simulink model "match_141121"  (R2018b)
settings: Solver=FixedStepDiscrete  StartTime=0.0  StopTime=1  RelTol=1e-3
undefined symbols (not defined in the file or in its folder): gray
libraries: hdlsllib x6, visionsources x1, dspmtrx3 x1
settings Model: Creator=Administrator  LastModifiedBy=Administrator
settings OptimizationCC: BlockReduction=off  ConditionallyExecuteInputs=off  DefaultParameterBehavior=Inlined
settings DebuggingCC: AlgebraicLoopMsg=error  SingleTaskRateTransMsg=error
settings HardwareCC: ProdBitPerPointer=32  ProdBitPerSizeT=32  ProdBitPerPtrDiffT=32  ProdLargestAtomicFloat=None  ProdIntDivRoundTo=Undefined  ProdEndianess=Unspecified  ProdWordSize=32  ProdHWDeviceType=ASIC/FPGA->ASIC/FPGA  TargetBitPerPointer=64  TargetBitPerSizeT=64  TargetBitPerPtrDiffT=64  TargetLongLongMode=on  TargetIntDivRoundTo=Zero  TargetEndianess=LittleEndian  TargetWordSize=64  TargetHWDeviceType=Custom Processor->MATLAB Host Computer  ProdEqTarget=off

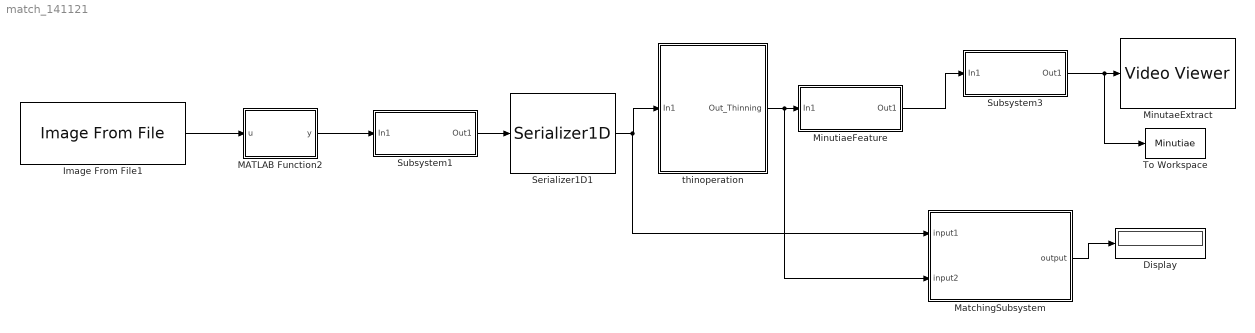
== system match_141121 ==
  Display : Display
  Image From File1 : visionsources/Image From File  Tag=vipblks_nd  FileName=C:\Users\Administrator\Desktop\chapter\101_4.tif  imagePorts=One multidimensional signal  Ts=0.1  ImageDataType=uint8  Signed=on  WordLength=16  sdImageDataType=uint(8)  FractionLengthMode=User-defined  FractionLength=15  OutPortLabels=R|G|B
      settings: SourceProductName=Computer Vision System Toolbox
  MATLAB Function2 : MATLAB Function  TreatAsAtomicUnit=on
  MatchingSubsystem : Subsystem
  MinutaeExtract : VideoViewer  colormapValue=gray(256)  FigPos=[1 1158 1920 1059]
  MinutiaeFeature : Subsystem  TreatAsAtomicUnit=on
  Serializer1D1 : hdlsllib/HDL Operations/Serializer1D  Ratio=1  IdleCycles=0  validIn=off  startOut=off  validOut=off  inputDataDimensions=8192  inputSampleTime=-1  inputSignalType=auto
      settings: SourceProductName=HDL Coder  SourceProductBaseCode=HD
  Subsystem1 : Subsystem
  Subsystem3 : Subsystem
  To Workspace : ToWorkspace  VariableName=Minutiae  SampleTime=-1
      settings: Save2DSignal=2-D array (concatenate along first dimension)
  thinoperation : Subsystem  TreatAsAtomicUnit=on
  wires:
  MATLAB Function2/1(y) -> Subsystem1/1(In1)
  Image From File1/1 -> MATLAB Function2/1(u)
  Subsystem1/1(Out1) -> Serializer1D1/1
  MinutiaeFeature/1(Out1) -> Subsystem3/1(In1)
  Subsystem3/1(Out1) -> To Workspace/1, MinutaeExtract/1
  Serializer1D1/1 -> MatchingSubsystem/1(input1), thinoperation/1(In1)
  thinoperation/1(Out_Thinning) -> MatchingSubsystem/2(input2), MinutiaeFeature/1(In1)
  MatchingSubsystem/1(output) -> Display/1

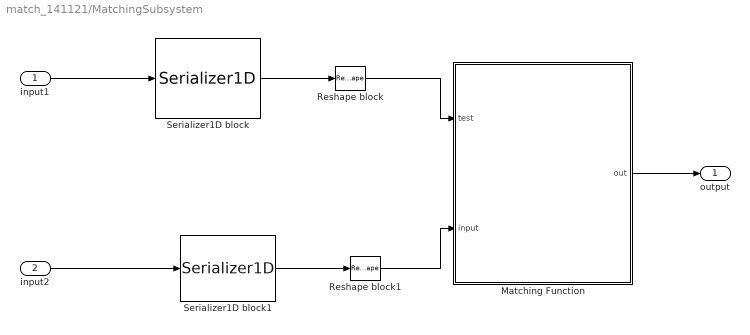
== system match_141121/MatchingSubsystem ==
  input1 : Inport
  input2 : Inport  Port=2
  Matching Function : MATLAB Function  TreatAsAtomicUnit=on
  Reshape block : Reshape  OutputDimensionality=Customize  OutputDimensions=[128,64]
  Reshape block1 : Reshape  OutputDimensionality=Customize  OutputDimensions=[128,64]
  Serializer1D block : hdlsllib/HDL Operations/Serializer1D  Ratio=1  IdleCycles=0  validIn=off  startOut=off  validOut=off  inputDataDimensions=8192  inputSampleTime=-1  inputSignalType=auto
      settings: SourceProductName=HDL Coder  SourceProductBaseCode=HD
  Serializer1D block1 : hdlsllib/HDL Operations/Serializer1D  Ratio=1  IdleCycles=0  validIn=off  startOut=off  validOut=off  inputDataDimensions=8192  inputSampleTime=-1  inputSignalType=auto
      settings: SourceProductName=HDL Coder  SourceProductBaseCode=HD
  output : Outport
  wires:
  Matching Function/1(out) -> output/1
  Serializer1D block/1 -> Reshape block/1
  Reshape block/1 -> Matching Function/1(test)
  input1/1 -> Serializer1D block/1
  Reshape block1/1 -> Matching Function/2(input)
  Serializer1D block1/1 -> Reshape block1/1
  input2/1 -> Serializer1D block1/1

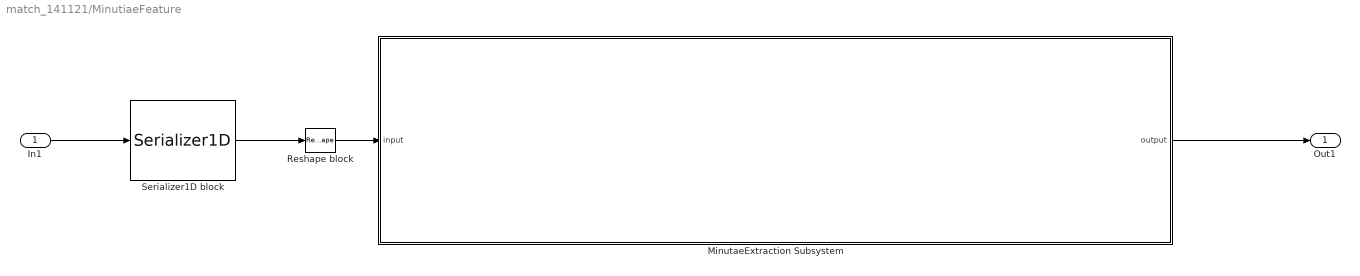
== system match_141121/MinutiaeFeature ==
  In1 : Inport
  MinutaeExtraction Subsystem : Subsystem  TreatAsAtomicUnit=on
  Reshape block : Reshape  OutputDimensionality=Customize  OutputDimensions=[128,64]
  Serializer1D block : hdlsllib/HDL Operations/Serializer1D  Ratio=1  IdleCycles=0  validIn=off  startOut=off  validOut=off  inputDataDimensions=8192  inputSampleTime=-1  inputSignalType=auto
      settings: SourceProductName=HDL Coder  SourceProductBaseCode=HD
  Out1 : Outport
  wires:
  In1/1 -> Serializer1D block/1
  MinutaeExtraction Subsystem/1(output) -> Out1/1
  Reshape block/1 -> MinutaeExtraction Subsystem/1(input)
  Serializer1D block/1 -> Reshape block/1

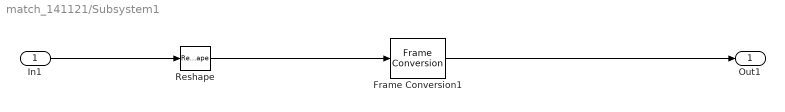
== system match_141121/Subsystem1 ==
  In1 : Inport
  Frame Conversion1 : FrameConversion  OutFrame=Sample-based
  Reshape : Reshape
  Out1 : Outport
  wires:
  Frame Conversion1/1 -> Out1/1
  Reshape/1 -> Frame Conversion1/1
  In1/1 -> Reshape/1

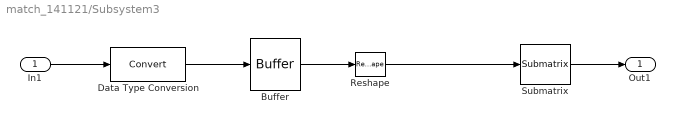
== system match_141121/Subsystem3 ==
  In1 : Inport
  Buffer : Buffer  N=8192  OutputFrames=off
  Data Type Conversion : DataTypeConversion
  Reshape : Reshape  OutputDimensionality=Customize  OutputDimensions=[128,64]
  Submatrix : dspmtrx3/Submatrix  RowSpan=Range of rows  RowStartMode=First  RowStartIndex=1  RowEndMode=Last  RowEndIndex=1  ColSpan=Range of columns  ColStartMode=First  ColStartIndex=1  ColEndMode=Last  ColEndIndex=1
  Out1 : Outport
  wires:
  Data Type Conversion/1 -> Buffer/1
  Buffer/1 -> Reshape/1
  Reshape/1 -> Submatrix/1
  Submatrix/1 -> Out1/1
  In1/1 -> Data Type Conversion/1

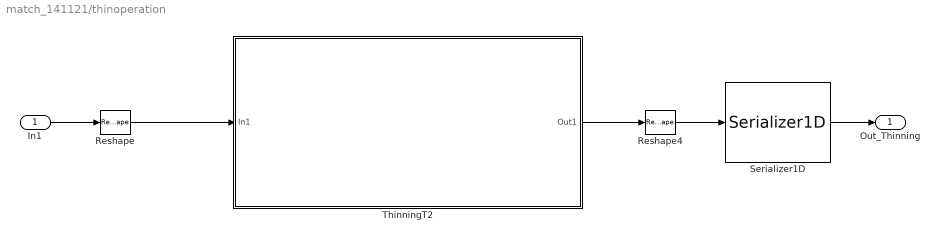
== system match_141121/thinoperation ==
  In1 : Inport
  Reshape : Reshape  OutputDimensionality=Customize  OutputDimensions=[128,64]
  Reshape4 : Reshape  OutputDimensionality=Column vector (2-D)  OutputDimensions=[128,64]
  Serializer1D : hdlsllib/HDL Operations/Serializer1D  Ratio=1  IdleCycles=0  validIn=off  startOut=off  validOut=off  inputDataDimensions=-1  inputSampleTime=-1  inputSignalType=auto
      settings: SourceProductName=HDL Coder  SourceProductBaseCode=HD
  ThinningT2 : Subsystem  TreatAsAtomicUnit=on
  Out_Thinning : Outport
  wires:
  ThinningT2/1(Out1) -> Reshape4/1
  Reshape/1 -> ThinningT2/1(In1)
  Serializer1D/1 -> Out_Thinning/1
  In1/1 -> Reshape/1
  Reshape4/1 -> Serializer1D/1

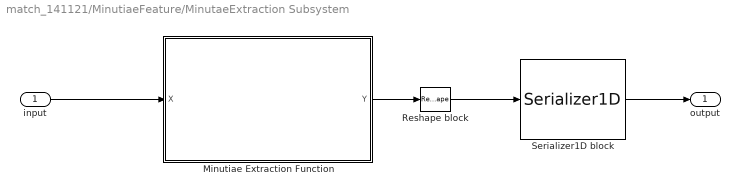
== system match_141121/MinutiaeFeature/MinutaeExtraction Subsystem ==
  input : Inport
  Minutiae Extraction Function : MATLAB Function  TreatAsAtomicUnit=on
  Reshape block : Reshape  OutputDimensionality=Column vector (2-D)  OutputDimensions=[128,64]
  Serializer1D block : hdlsllib/HDL Operations/Serializer1D  Ratio=8192  IdleCycles=0  validIn=off  startOut=off  validOut=off  inputDataDimensions=-1  inputSampleTime=-1  inputSignalType=auto
      settings: SourceProductName=HDL Coder  SourceProductBaseCode=HD
  output : Outport
  wires:
  input/1 -> Minutiae Extraction Function/1(X)
  Serializer1D block/1 -> output/1
  Minutiae Extraction Function/1(Y) -> Reshape block/1
  Reshape block/1 -> Serializer1D block/1

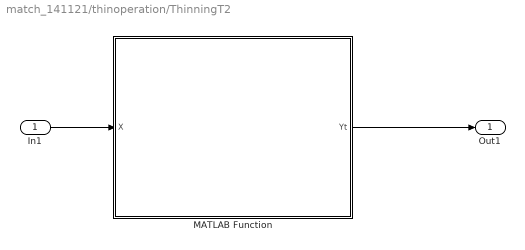
== system match_141121/thinoperation/ThinningT2 ==
  In1 : Inport
  MATLAB Function : MATLAB Function  TreatAsAtomicUnit=on
  Out1 : Outport
  wires:
  In1/1 -> MATLAB Function/1(X)
  MATLAB Function/1(Yt) -> Out1/1

== matlab function match_141121/MATLAB Function2 ==
  data: u input; y output
function y = fcn(u)
%#codegen
%i = rgb2gray(u);
b = u(100:227,150:213);
y = imbinarize(b);
%y = y(100:227,150:213);
%y = imbinarize(r);

== matlab function match_141121/thinoperation/ThinningT2/MATLAB Function ==
  data: X input; Yt output
function Yt=thinningTh(X)
%img = imread ('2_4.jpg'); 
%Xr = rgb2gray(img);
%%%X = imbinarize(Xr);
%X = X(1:128,1:64);
[M,N]=size(X);
Yt = false(M,N);
Y=false(M,N,20);
Z=false(M,N,20);
Y(:,:,1)=X;
Z(:,:,1)=X;
for k=2:20
    Y(:,:,k)=Y(:,:,k-1);
    for i=2:M-1
        for j=2:N-1
            y11=Y(i-1,j-1,k);
            y12=Y(i-1,j,k);
            y13=Y(i-1,j+1,k);
            y21=Y(i,j-1,k);
            y22=Y(i,j,k);
            y23=Y(i,j+1,k);
            y31=Y(i+1,j-1,k);
            y32=Y(i+1,j,k);
            y33=Y(i+1,j+1,k);
            if y22==0
                if y11==1&&y12==1&&y13==1&&y31==0&&y32==0&&y33==0
                    Y(i,j,k)=1;
                elseif y11==1&&y13==0&&y21==1&&y23==0&&y31==1&&y33==0
                    Y(i,j,k)=1;
                elseif y11==0&&y12==0&&y13==0&&y31==1&&y32==1&&y33==1
                    Y(i,j,k)=1;
                elseif y11==0&&y13==1&&y21==0&&y23==1&&y31==0&&y33==1
                    Y(i,j,k)=1;
                elseif y12==1&&y13==1&&y21==0&&y23==1&&y32==0
                    Y(i,j,k)=1;
                elseif y11==1&&y12==1&&y21==1&&y23==0&&y32==0
                    Y(i,j,k)=1;
                elseif y12==0&&y21==1&&y23==0&&y31==1&&y21==1
                    Y(i,j,k)=1;
                elseif y12==0&&y21==0&&y23==1&&y32==1&&y33==1
                    Y(i,j,k)=1;
                    %extra
                elseif y11==0&&y12==0&&y23==1&&y31==1&&y32==1&&y33==1
                    Y(i,j,k)=1;
                end
            else
            end
        end
    end
%    Y(:,:,k)= Y(:,:,k-1);
     if Y(:,:,k)==Y(:,:,k-1)
%         break;
     end
end
Yt=Y(:,:,k);
%figure;
%imshow(Y);

== matlab function match_141121/MatchingSubsystem/Matching Function ==
  data: test input; out output; input input
function out = match(test, input)
%test = zeros(rows,col);
%input = zeros(rows,col);
%[row,col]= size(input);
test = uint8(test);
input = uint8(input);
for i=1:128
    for j=1:64
        %input(i,j);
        if test == input
            out = 1;
        else
            out = 0;
        end
    end
end
end

== matlab function match_141121/MinutiaeFeature/MinutaeExtraction Subsystem/Minutiae Extraction Function ==
  data: X input; Y output
function Y=minuextractT(X)
%img = imread ('101_7.tif'); 
%Xr = rgb2gray(img);
%Xt = imbinarize(img);
%X=~bwmorph(Xt,'thin',Inf);
[M,N]=size(X);
%mi(:,:)=X;
Y=false(M,N);
Y(:,:)=X;
%[M,N]=size(X);
mi=false(M,N);

for i=2:M-1
    for j=2:N-1
        % * * * y11 y12 y13
        % * @ * y21 y22 y23
        % * * * y31 y32 y33
        y11=Y(i-1,j-1);
        y12=Y(i-1,j);
        y13=Y(i-1,j+1);
        y21=Y(i,j-1);
        y22=Y(i,j);
        y23=Y(i,j+1);
        y31=Y(i+1,j-1);
        y32=Y(i+1,j);
        y33=Y(i+1,j+1);
        if y22==0
            if y11+y12+y13+y23+y33+y31+y21+y32==7
                mi(i,j)=1;
            elseif y11==0 && y12==1 && y13==0 && y21==1 && y23==1 && y31==1 && y32==0 && y33==1
                mi(i,j)=2;
            elseif y11==1 && y12==0 && y13==1 && y21==1 && y23==1 && y31==0 && y32==1 && y33==0
                mi(i,j)=2;
            elseif y11==0 && y12==1 && y13==1 && y21==1 && y23==0 && y31==0 && y32==1 && y33==1
                mi(i,j)=2;
            elseif y11==1 && y12==1 && y13==0 && y21==0 && y23==1 && y31==1 && y32==1 && y33==0
                mi(i,j)=2;
            elseif y11==1 && y12==0 && y13==1 && y21==0 && y23==0 && y31==1 && y32==1 && y33==1
                mi(i,j)=2;
            elseif y11==1 && y12==1 && y13==1 && y21==0 && y23==0 && y31==1 && y32==0 && y33==1
                mi(i,j)=2;
            elseif y11==1 && y12==0 && y13==1 && y21==0 && y23==1 && y31==1 && y32==0 && y33==1
                mi(i,j)=2;
            elseif y11==1 && y12==0 && y13==1 && y21==1 && y23==0 && y31==1 && y32==0 && y33==1
                mi(i,j)=2;
            elseif y11==0 && y12==1 && y13==0 && y21==1 && y23==1 && y31==0 && y32==1 && y33==1
                mi(i,j)=2;
            elseif y11==0 && y12==1 && y13==1 && y21==1 && y23==1 && y31==0 && y32==1 && y33==0
                mi(i,j)=2;
            elseif y11==0 && y12==1 && y13==0 && y21==1 && y23==1 && y31==1 && y32==1 && y33==0
                mi(i,j)=2;
            elseif y11==1 && y12==1 && y13==0 && y21==1 && y23==1 && y31==0 && y32==1 && y33==0
                mi(i,j)=2;
            elseif y11==1 && y12==0 && y13==1 && y21==0 && y23==0 && y31==0 && y32==1 && y33==1
                mi(i,j)=2;
            elseif y11==1 && y12==0 && y13==1 && y21==0 && y23==0 && y31==1 && y32==1 && y33==0
                mi(i,j)=2;
            elseif y11==0 && y12==1 && y13==1 && y21==0 && y23==0 && y31==1 && y32==0 && y33==1
                mi(i,j)=2;
            elseif y11==1 && y12==1 && y13==0 && y21==0 && y23==0 && y31==1 && y32==0 && y33==1
                mi(i,j)=2;
            elseif y11==1 && y12==1 && y13==0 && y21==0 && y23==1 && y31==1 && y32==0 && y33==1
                mi(i,j)=2;
            elseif y11==1 && y12==0 && y13==1 && y21==1 && y23==0 && y31==0 && y32==1 && y33==1
                mi(i,j)=2;
            elseif y11==1 && y12==0 && y13==1 && y21==0 && y23==1 && y31==1 && y32==1 && y33==0
                mi(i,j)=2;
            elseif y11==0 && y12==1 && y13==1 && y21==1 && y23==0 && y31==1 && y32==0 && y33==1
                mi(i,j)=2;
            elseif y11==1 && y12==0 && y13==1 && y21==1 && y23==0 && y31==0 && y32==0 && y33==1
                mi(i,j)=2;
            elseif y11==0 && y12==0 && y13==1 && y21==1 && y23==0 && y31==1 && y32==0 && y33==1
                mi(i,j)=2;
            elseif y11==1 && y12==0 && y13==0 && y21==0 && y23==1 && y31==1 && y32==0 && y33==1
                mi(i,j)=2;
            elseif y11==1 && y12==0 && y13==1 && y21==0 && y23==1 && y31==1 && y32==0 && y33==0
                mi(i,j)=2;
            end
        else
        end
    end
end
 Y=mi(:,:);

% %false minutiae deletion
% for M=1:300
%     for N=1:200
%         if mi(M,N)==1||mi(M,N)==2
%             d=20;
%             if M<d||M+d>300||N<d||N+d>200
%                 mi(M,N)=0;
%             else
%             end
%         else
%         end
%     end
% end
% 
% for N=1:200
%     for M=1:300
%         if mi(M,N)==1||mi(M,N)==2
%             for i=1:300
%                 for j=1:200
%                     if mi(i,j)==1||mi(i,j)==2
%                         if mi(M,N)==mi(i,j)
%                             d=10;
%                         else
%                             d=5;
%                         end
%                         a=sqrt((M-i)^2+(N-j)^2);
%                         if a<d&&a>0
%                             mi(M,N)=0;
%                             mi(i,j)=0;
%                         else
%                         end
%                     end
%                 end
%             end
%         else
%         end
%     end
% end
% figure
% hold on
% for M=1:320
%     for N=1:240
%         if mi(M,N)==1
%             a=round((M-1)/12)+1;
%             b=round((N-1)/12)+1;
%             plot(1*(N++1i*(M)),'ro','LineWidth',2)
%         elseif mi(M,N)==2
%             a=round((M-1)/12)+1;
%             b=round((N-1)/12)+1;
%             plot(1*(N++1i*(M)),'bo','LineWidth',2)
%         end
%     end
% end

%figure;imshow(img);
%figure;imshow(Xr);
%figure;imshow(Xt);
%figure;imshow(X);
%figure;imshow(Y);
